simulink model "ssc_bridge_rectifier"  (R2014a)
settings: Solver=ode113  StartTime=0.0  StopTime=0.05  MaxStep=0.001  RelTol=1e-3
libraries: fl_lib x11, nesl_utility x2
Description:
  | Full-Wave Bridge Rectifier
  | 
  | This example shows an ideal AC transformer plus full-wave bridge rectifier.
  | It converts 120 volts AC to 12 volts DC. The transformer has a turns ratio
  | of 14, stepping the supply down to 8.6 volts rms, i.e. 8.6*sqrt(2) = 12 volts
  | pk-pk. The full-wave bridge rectifier plus capacitor combination
  | then converts this to DC. The resistor represents a typical load.
  | 
  | The model can be used to size the capacitor required for a specified load.
  | For a given size of capacitor, as the load resistance is increased, the ripple
  | in the DC voltage increases. The model can also be used to drive an
  | application circuit in order to assess the effect of the ripple.
  | 
  | 
  | 
  | 
  | Copyright 2008-2014 The MathWorks, Inc.
settings Model: ExtModeAutoUpdateStatusClock=off  Creator=MathWorks  LastModifiedBy=User
settings DataIOCC: SignalLoggingSaveFormat=ModelDataLogs
settings OptimizationCC: ExpressionDepthLimit=2147483647  InitFltsAndDblsToZero=on  EfficientMapNaN2IntZero=off
settings DebuggingCC: SaveWithParameterizedLinksMsg=none  UnderspecifiedInitializationDetection=Classic  SignalResolutionControl=TryResolveAllWithWarning  FcnCallInpInsideContextMsg=UseLocalSettings  StateNameClashWarn=warning
settings GRTTargetCC: TargetFcnLib=ansi_tfl_tmw.mat  CombineOutputUpdateFcns=off  GRTInterface=on
settings SimscapeCC: ExplicitSolverDiagnosticOptions=none

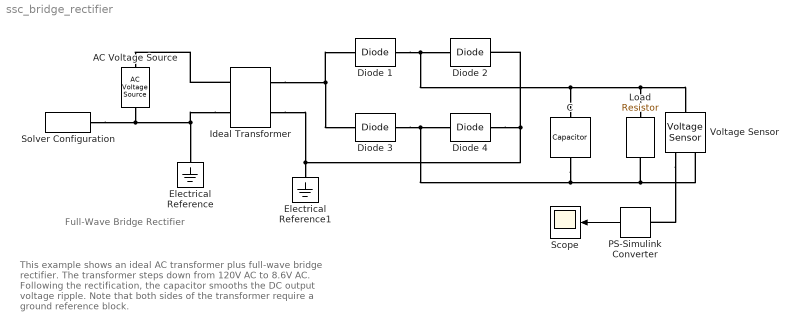
== system ssc_bridge_rectifier ==
  note: This example shows an ideal AC transformer plus
      | full-wave bridge rectifier. The transformer steps
      | down from 120V AC to 8.6V AC. Following the rectification,
      | the capacitor smooths the DC output voltage ripple. Note
      | that both sides of the transformer require a ground
      | reference block.
  note: Full-Wave Bridge Rectifier
  AC Voltage Source : fl_lib/Electrical/Electrical Sources/AC Voltage Source  amp=sqrt(2)*120 V  shift=0 deg  frequency=60 Hz  omega=0 rad/s
  C : fl_lib/Electrical/Electrical Elements/Capacitor  c=470e-06 F  r=1e-06 Ohm  g=0 1/Ohm  i_specify=off  i_priority=High  i=0 A  v_specify=off  v_priority=High  v=0 V  vc_specify=on  vc_priority=High  vc=0 V
  Diode {1..4} (4 alike) : fl_lib/Electrical/Electrical Elements/Diode  Vf=0.6 V  Ron=0.3 Ohm  Goff=1e-08 1/Ohm  i_specify=off  i_priority=High  i=0 A  v_specify=off  v_priority=High  v=0 V
  Electrical Reference : fl_lib/Electrical/Electrical Elements/Electrical Reference
  Electrical Reference1 : fl_lib/Electrical/Electrical Elements/Electrical Reference
  Ideal Transformer : fl_lib/Electrical/Electrical Elements/Ideal Transformer  n=14  i1_specify=off  i1_priority=High  i1=0 A  v1_specify=off  v1_priority=High  v1=0 V  i2_specify=off  i2_priority=High  i2=0 A  v2_specify=off  v2_priority=High  v2=0 V
  Load : fl_lib/Electrical/Electrical Elements/Resistor  R=100 Ohm  i_specify=off  i_priority=High  i=0 A  v_specify=off  v_priority=High  v=0 V
  PS-Simulink Converter : nesl_utility/PS-Simulink Converter  PhysicalDomain=network_engine_domain  SubClassName=ps_output  LeftPortType=input  RightPortType=output  PseudoPeriodic=off  Frequencies=[]  Unit=1  AffineConversion=off
  Scope : Scope
      settings: YMin=0  YMax=20
  Solver Configuration : nesl_utility/Solver Configuration  PhysicalDomain=network_engine_domain  SubClassName=solver  LeftPortType=input  RightPortType=generic  Accelerate=off  Tones=[]  Harmonics=[]  SimulateNoise=off  Profile=off  UseLocalSampling=off  EnableSwitchedLinearOptims=on  FrequencyDomain=off  UseCCode=off  RelTol=0.001  AbsTol=1e-06  MinStep=1e-09  ToWorkspace=off  DoDC=off  ResidualTolerance=1e-9  UseLocalSolver=off  LocalSolverChoice=NE_BACKWARD_EULER_ADVANCER  LocalSolverSampleTime=.001  DoFixedCost=off  MaxNonlinIter=3  MaxModeIter=2  LinearAlgebra=Sparse  DelaysMemoryBudget=1024  AutomaticFiltering=on  FilteringTimeConstant=0.001
  Voltage Sensor : fl_lib/Electrical/Electrical Sensors/Voltage Sensor
  wires:
  PS-Simulink Converter/1 -> Scope/1
  connections:
  Ideal Transformer/LConn2 -- AC Voltage Source/RConn1 -- Solver Configuration/RConn1 -- Electrical Reference/LConn1
  Ideal Transformer/LConn1 -- AC Voltage Source/LConn1
  Ideal Transformer/RConn1 -- Diode 3/RConn1 -- Diode 1/LConn1
  Diode 1/RConn1 -- Diode 2/RConn1 -- Voltage Sensor/LConn1 -- Load/LConn1 -- C/LConn1
  Diode 3/LConn1 -- Diode 4/LConn1 -- Voltage Sensor/RConn2 -- Load/RConn1 -- C/RConn1
  Ideal Transformer/RConn2 -- Diode 2/LConn1 -- Diode 4/RConn1 -- Electrical Reference1/LConn1
  Voltage Sensor/RConn1 -- PS-Simulink Converter/LConn1
